simulink model "sim_embedded_kalman"  (R2024b)
settings: Solver=ode4  StartTime=t_0  StopTime=t_f  FixedStep=dt  RelTol=1e-8
undefined symbols (not defined in the file or in its folder): airdata, atm_poly, GROUND_LEVEL, kalm_gain, kalm_initial_state, kalm_measure_matrix, kalm_sample_rate, kalm_state_matrix
libraries: simulink x1
settings Model: SimulationMode=accelerator  Creator=yevge  LastModifiedBy=Aiden Gaydos
settings DebuggingCC: AlgebraicLoopMsg=error  CheckMatrixSingularityMsg=error

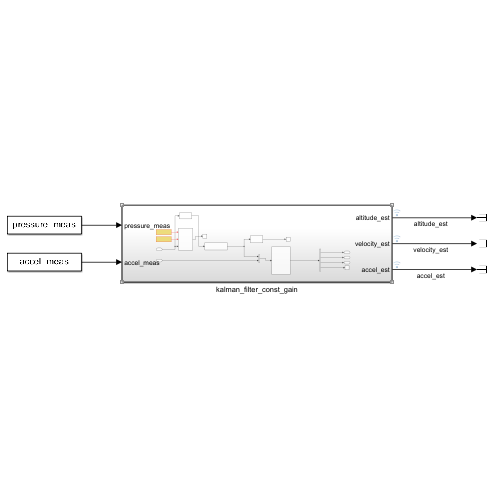
[thumbnail: Simulink's stored preview of the top-level diagram]
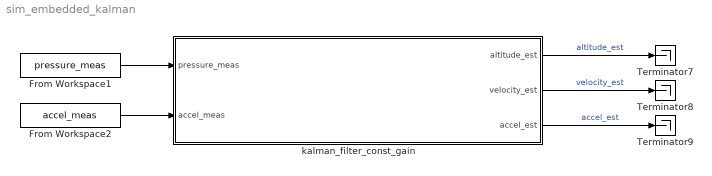
== system sim_embedded_kalman ==
  From Workspace1 : FromWorkspace  VariableName=pressure_meas
  From Workspace2 : FromWorkspace  VariableName=accel_meas
  Terminator7 : Terminator
  Terminator8 : Terminator
  Terminator9 : Terminator
  kalman_filter_const_gain : Subsystem
  wires:
  kalman_filter_const_gain/1(altitude_est) -> Terminator7/1  "altitude_est"
  kalman_filter_const_gain/2(velocity_est) -> Terminator8/1  "velocity_est"
  kalman_filter_const_gain/3(accel_est) -> Terminator9/1  "accel_est"
  From Workspace2/1 -> kalman_filter_const_gain/2(accel_meas)
  From Workspace1/1 -> kalman_filter_const_gain/1(pressure_meas)

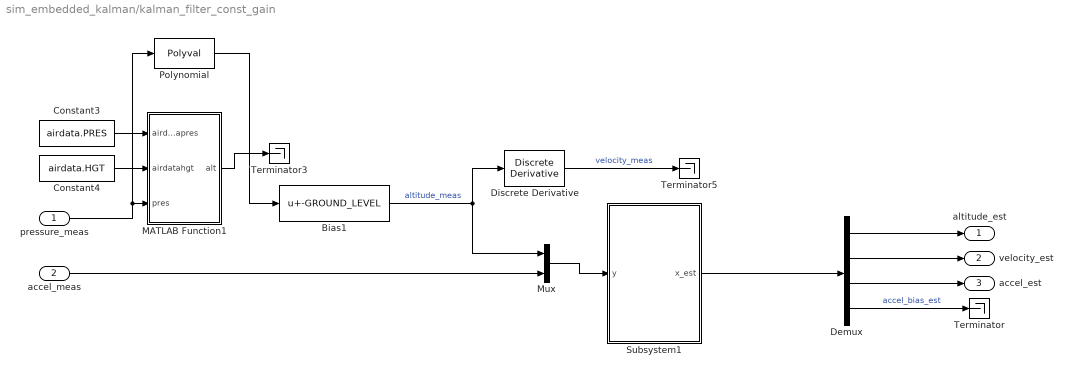
== system sim_embedded_kalman/kalman_filter_const_gain ==
  pressure_meas : Inport
  accel_meas : Inport  Port=2
  Bias1 : Bias  Bias=-GROUND_LEVEL  SaturateOnIntegerOverflow=off
  Constant3 : Constant  Value=airdata.PRES
  Constant4 : Constant  Value=airdata.HGT
  Demux : Demux
  Discrete Derivative : simulink/Discrete/Discrete Derivative  gainval=1  ICPrevScaledInput=0.0  OutMin=[]  OutMax=[]  OutDataType=fixdt(1, 16)  OutScaling=2^-10  DoSatur=off
  MATLAB Function1 : MATLAB Function  TreatAsAtomicUnit=on
  Mux : Mux  Inputs=2
  Polynomial : Polyval  Coefs=atm_poly
  Subsystem1 : Subsystem
  Terminator : Terminator
  Terminator3 : Terminator
  Terminator5 : Terminator
  altitude_est : Outport  PortDimensions=1
  velocity_est : Outport  Port=2  PortDimensions=1
  accel_est : Outport  Port=3  PortDimensions=1
  wires:
  Demux/4 -> Terminator/1  "accel_bias_est"
  Demux/3 -> accel_est/1
  Demux/2 -> velocity_est/1
  Demux/1 -> altitude_est/1
  Bias1/1 -> Mux/1, Discrete Derivative/1  "altitude_meas"
  pressure_meas/1 -> Polynomial/1, MATLAB Function1/3(pres)
  Mux/1 -> Subsystem1/1(y)
  accel_meas/1 -> Mux/2
  Subsystem1/1(x_est) -> Demux/1
  Constant4/1 -> MATLAB Function1/2(airdatahgt)
  Discrete Derivative/1 -> Terminator5/1  "velocity_meas"
  Polynomial/1 -> Bias1/1
  Constant3/1 -> MATLAB Function1/1(airdatapres)
  MATLAB Function1/1(alt) -> Terminator3/1

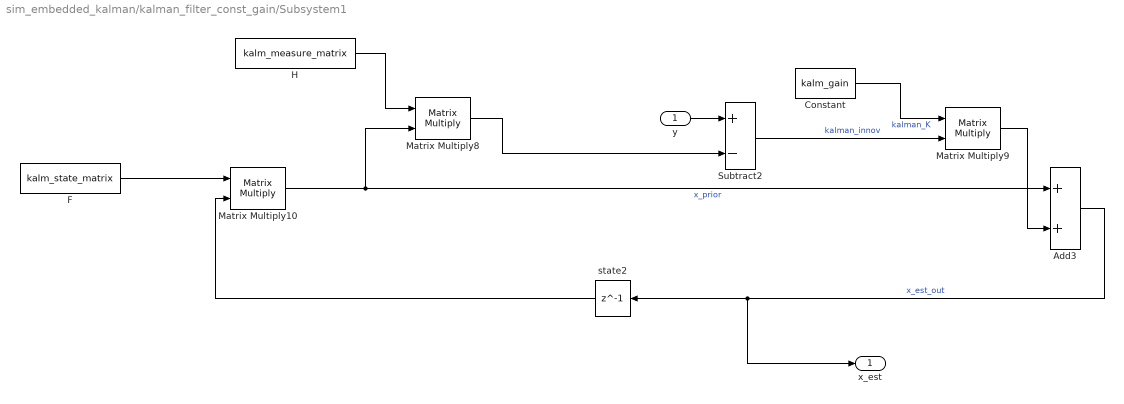
== system sim_embedded_kalman/kalman_filter_const_gain/Subsystem1 ==
  y : Inport  SampleTime=1/kalm_sample_rate
  Add3 : Sum
  Constant : Constant  Value=kalm_gain
  F : Constant  Value=kalm_state_matrix
  H : Constant  Value=kalm_measure_matrix
  Matrix Multiply10 : Product  Multiplication=Matrix(*)
  Matrix Multiply8 : Product  Multiplication=Matrix(*)
  Matrix Multiply9 : Product  Multiplication=Matrix(*)
  Subtract2 : Sum  Inputs=+-
  state2 : Delay  DelayLength=1  InitialCondition=kalm_initial_state  SampleTime=1/kalm_sample_rate
  x_est : Outport  SampleTime=1/kalm_sample_rate
  wires:
  Matrix Multiply10/1 -> Matrix Multiply8/2, Add3/1  "x_prior"
  y/1 -> Subtract2/1
  Matrix Multiply9/1 -> Add3/2
  Constant/1 -> Matrix Multiply9/1  "kalman_K"
  Subtract2/1 -> Matrix Multiply9/2  "kalman_innov"
  Matrix Multiply8/1 -> Subtract2/2
  F/1 -> Matrix Multiply10/1
  H/1 -> Matrix Multiply8/1
  Add3/1 -> x_est/1, state2/1  "x_est_out"
  state2/1 -> Matrix Multiply10/2

== matlab function sim_embedded_kalman/kalman_filter_const_gain/MATLAB Function1 ==
  data: airdatapres input; airdatahgt input; pres input; alt output
function alt = pres_to_alt(airdatapres,airdatahgt,pres)
    alt = double(interp1(airdatapres,airdatahgt,pres,"linear","extrap"));
end
